simulink model "gait_recorder"  (R2015b)
settings: Solver=FixedStepDiscrete  StartTime=0.0  StopTime=inf  FixedStep=.0001  RelTol=1e-3
libraries: xpcethercatlib x14, slrtlib x8
settings Model: xpc_rtwmakecfg_data=_xpcethercatlib_  SimulationMode=external  Creator=rtheyyun  LastModifiedBy=rafae
settings SolverCC: EnableConcurrentExecution=on  ConcurrentTasks=on
settings DataIOCC: SaveFinalState=on  SaveFormat=StructureWithTime  SignalLoggingSaveFormat=ModelDataLogs  InspectSignalLogs=on
settings OptimizationCC: BlockReduction=off  OptimizeBlockIOStorage=off  BufferReuse=off  GlobalBufferReuse=off  ExpressionFolding=off  ExpressionDepthLimit=2147483647  LocalBlockOutputs=off
settings DebuggingCC: ReadBeforeWriteMsg=DisableAll  WriteAfterWriteMsg=DisableAll  WriteAfterReadMsg=DisableAll  UnderspecifiedInitializationDetection=Classic  MergeDetectMultiDrivingBlocksExec=none  SolverPrmCheckMsg=warning  InheritedTsInSrcMsg=none  FcnCallInpInsideContextMsg=UseLocalSettings  StateNameClashWarn=warning
settings HardwareCC: ProdBitPerPointer=32  ProdLargestAtomicFloat=None  ProdWordSize=32  ProdLongLongMode=on  ProdHWDeviceType=Generic->32-bit x86 compatible
settings RTWCC: SystemTargetFile=slrt.tlc  TemplateMakefile=slrt_default_tmf  Description=Simulink Real-Time  RTWVerbose=off  RTWCompilerOptimization=on
settings SimulinkRealTimeCC: GeneratePreprocessorConditionals=Disable all  xPCisModelTimeout=off  xPCModelTimeoutSecs=20  xPCConcurrentTasks=on
settings ConfigComp: CovModelRefEnable=Off  CovSFcnEnable=off

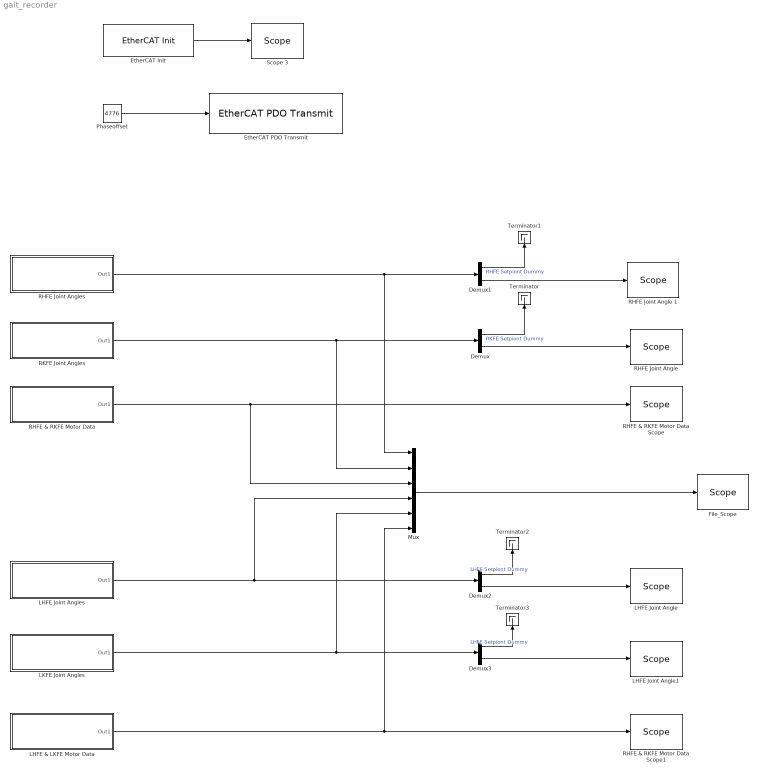
== system gait_recorder ==
  Demux{,1..3} (4 alike) : Demux  Outputs=2
  "EtherCAT Init " : xpcethercatlib/EtherCAT Init   Priority=0  config_file=C:\Users\rafae\Documents\GitHub\simulink-models\EtherCAT Config files\quad_slave_both_legs_v1.0.xml  device_id=0  pci_bus=2  pci_slot=0  dctuning=2  enaDebug=off  enaDC=off  errLink=on  masterDbg=on  stateChgDbg=on  baseClock=off  masterCfg=on  logFile='c:\dbglog.txt'  sample_time=0.001000
  "EtherCAT PDO Transmit " : xpcethercatlib/EtherCAT PDO Transmit   Priority=3  sig_name=RHFE.Outputs.jointSetpoint  sig_offset=12496  sig_type=uint32  type_size=32  sig_dim=1  device_id=0  sample_time=0.001000
  File_Scope : slrtlib/Displays and Logging/Scope   scopeno=8  scopetype=File  autostart=on  viewmode=Graphical sliding  formatstr='%15.6f'  grid=on  ylimits=[0,0]  nosamples=50000  noprepostsamples=0  interleave=1  triggermode=FreeRun  triggersignal=1  trigsignalfromport=off  triggerlevel=0.0  triggerslope=Either  triggerscope=1  triggersample=0  filename=gait.dat  mode=Lazy  writesize=512  autorestart=on  dynamicfilemode=off  maxwritefilesize=512*1024^2
  LHFE & LKFE Motor Data : Subsystem
  LHFE Joint Angle : slrtlib/Displays and Logging/Scope   scopeno=2  scopetype=Target  autostart=on  viewmode=Graphical sliding  formatstr='%15.6f'  grid=on  ylimits=[0,0]  nosamples=50000  noprepostsamples=0  interleave=1  triggermode=FreeRun  triggersignal=1  trigsignalfromport=off  triggerlevel=0.0  triggerslope=Either  triggerscope=1  triggersample=0  filename=data.dat  mode=Lazy  writesize=512  autorestart=off  dynamicfilemode=off  maxwritefilesize=512*1024^2
  LHFE Joint Angle1 : slrtlib/Displays and Logging/Scope   scopeno=5  scopetype=Target  autostart=on  viewmode=Graphical sliding  formatstr='%15.6f'  grid=on  ylimits=[0,0]  nosamples=50000  noprepostsamples=0  interleave=1  triggermode=FreeRun  triggersignal=1  trigsignalfromport=off  triggerlevel=0.0  triggerslope=Either  triggerscope=1  triggersample=0  filename=data.dat  mode=Lazy  writesize=512  autorestart=off  dynamicfilemode=off  maxwritefilesize=512*1024^2
  LHFE Joint Angles : Subsystem
  LKFE Joint Angles : Subsystem
  Mux : Mux  Inputs=6
  Phaseoffset : Constant  Value=4776  OutDataTypeStr=uint32
  RHFE & RKFE Motor Data : Subsystem
  RHFE & RKFE Motor Data Scope : slrtlib/Displays and Logging/Scope   scopeno=3  scopetype=Target  autostart=on  viewmode=Graphical sliding  formatstr='%15.6f'  grid=on  ylimits=[0,0]  nosamples=50000  noprepostsamples=0  interleave=1  triggermode=FreeRun  triggersignal=1  trigsignalfromport=off  triggerlevel=0.0  triggerslope=Either  triggerscope=1  triggersample=0  filename=data.dat  mode=Lazy  writesize=512  autorestart=off  dynamicfilemode=off  maxwritefilesize=512*1024^2
  RHFE & RKFE Motor Data Scope1 : slrtlib/Displays and Logging/Scope   scopeno=6  scopetype=Target  autostart=on  viewmode=Graphical sliding  formatstr='%15.6f'  grid=on  ylimits=[0,0]  nosamples=50000  noprepostsamples=0  interleave=1  triggermode=FreeRun  triggersignal=1  trigsignalfromport=off  triggerlevel=0.0  triggerslope=Either  triggerscope=1  triggersample=0  filename=data.dat  mode=Lazy  writesize=512  autorestart=off  dynamicfilemode=off  maxwritefilesize=512*1024^2
  "RHFE Joint Angle " : slrtlib/Displays and Logging/Scope   scopeno=4  scopetype=Target  autostart=on  viewmode=Graphical sliding  formatstr='%15.6f'  grid=on  ylimits=[0,0]  nosamples=50000  noprepostsamples=0  interleave=1  triggermode=FreeRun  triggersignal=1  trigsignalfromport=off  triggerlevel=0.0  triggerslope=Either  triggerscope=1  triggersample=0  filename=data.dat  mode=Lazy  writesize=512  autorestart=off  dynamicfilemode=off  maxwritefilesize=512*1024^2
  RHFE Joint Angle 1 : slrtlib/Displays and Logging/Scope   scopeno=1  scopetype=Target  autostart=on  viewmode=Graphical sliding  formatstr='%15.6f'  grid=on  ylimits=[0,0]  nosamples=50000  noprepostsamples=0  interleave=1  triggermode=FreeRun  triggersignal=1  trigsignalfromport=off  triggerlevel=0.0  triggerslope=Either  triggerscope=1  triggersample=0  filename=data.dat  mode=Lazy  writesize=512  autorestart=off  dynamicfilemode=off  maxwritefilesize=512*1024^2
  RHFE Joint Angles : Subsystem
  RKFE Joint Angles : Subsystem
  Scope 3 : slrtlib/Displays and Logging/Scope   scopeno=7  scopetype=Target  autostart=on  viewmode=Numerical  formatstr='%15.6f'  grid=on  ylimits=[0,0]  nosamples=3  noprepostsamples=0  interleave=1  triggermode=FreeRun  triggersignal=1  trigsignalfromport=off  triggerlevel=0.0  triggerslope=Either  triggerscope=1  triggersample=0  filename=data.dat  mode=Lazy  writesize=512  autorestart=off  dynamicfilemode=off  maxwritefilesize=512*1024^2
  Terminator{,1..3} (4 alike) : Terminator
  wires:
  "EtherCAT Init "/1 -> Scope 3/1
  Phaseoffset/1 -> "EtherCAT PDO Transmit "/1
  RHFE Joint Angles/1(Out1) -> Mux/1, Demux1/1
  Demux/2 -> "RHFE Joint Angle "/1
  Demux/1 -> Terminator/1  "RKFE Setpiont Dummy"
  RKFE Joint Angles/1(Out1) -> Mux/2, Demux/1
  Demux1/2 -> RHFE Joint Angle 1/1
  Demux1/1 -> Terminator1/1  "RHFE Setpiont Dummy"
  Mux/1 -> File_Scope/1
  RHFE & RKFE Motor Data/1(Out1) -> RHFE & RKFE Motor Data Scope/1, Mux/3
  LHFE & LKFE Motor Data/1(Out1) -> RHFE & RKFE Motor Data Scope1/1, Mux/6
  LHFE Joint Angles/1(Out1) -> Demux2/1, Mux/4
  Demux2/2 -> LHFE Joint Angle/1
  Demux2/1 -> Terminator2/1  "LHFE Setpiont Dummy"
  LKFE Joint Angles/1(Out1) -> Mux/5, Demux3/1
  Demux3/2 -> LHFE Joint Angle1/1
  Demux3/1 -> Terminator3/1  "LHFE Setpiont Dummy"

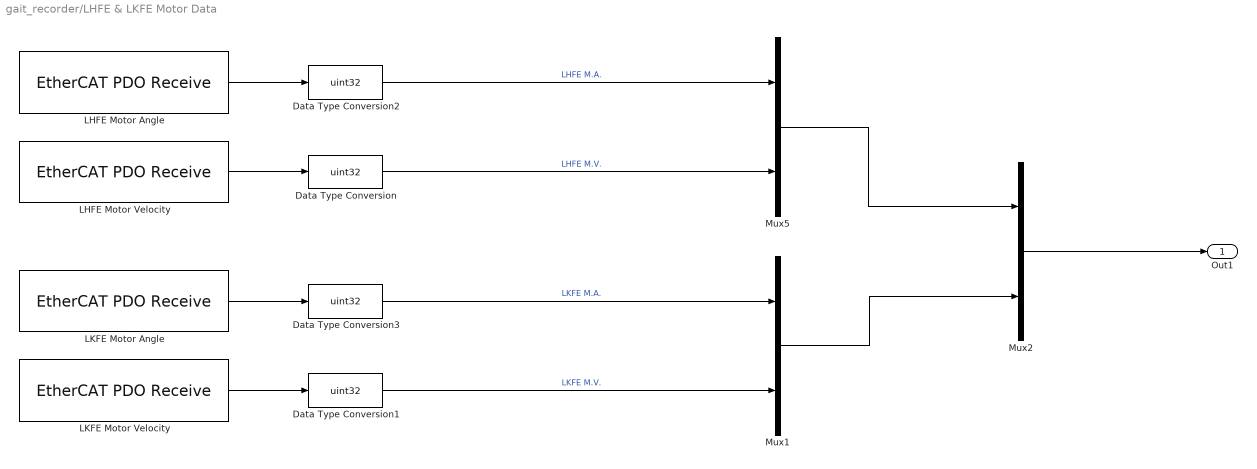
== system gait_recorder/LHFE & LKFE Motor Data ==
  Data Type Conversion{,1..3} (4 alike) : DataTypeConversion  OutDataTypeStr=uint32
  LHFE Motor Angle : xpcethercatlib/EtherCAT PDO Receive  Priority=2  sig_name=LHFE.Inputs.motorAngle  sig_offset=240  sig_type=uint16  type_size=16  sig_dim=1  device_id=0  sample_time=0.001000
  LHFE Motor Velocity : xpcethercatlib/EtherCAT PDO Receive  Priority=2  sig_name=LHFE.Inputs.motorVelocity  sig_offset=256  sig_type=int16  type_size=16  sig_dim=1  device_id=0  sample_time=0.001000
  LKFE Motor Angle : xpcethercatlib/EtherCAT PDO Receive  Priority=2  sig_name=LKFE.Inputs.motorAngle  sig_offset=528  sig_type=uint16  type_size=16  sig_dim=1  device_id=0  sample_time=0.001000
  LKFE Motor Velocity : xpcethercatlib/EtherCAT PDO Receive  Priority=2  sig_name=LKFE.Inputs.motorVelocity  sig_offset=544  sig_type=int16  type_size=16  sig_dim=1  device_id=0  sample_time=0.001000
  Mux1 : Mux  Inputs=2
  Mux2 : Mux  Inputs=2
  Mux5 : Mux  Inputs=2
  Out1 : Outport
  wires:
  Mux5/1 -> Mux2/1
  LHFE Motor Angle/1 -> Data Type Conversion2/1
  LHFE Motor Velocity/1 -> Data Type Conversion/1
  Mux1/1 -> Mux2/2
  Mux2/1 -> Out1/1
  LKFE Motor Angle/1 -> Data Type Conversion3/1
  LKFE Motor Velocity/1 -> Data Type Conversion1/1
  Data Type Conversion/1 -> Mux5/2  "LHFE M.V."
  Data Type Conversion1/1 -> Mux1/2  "LKFE M.V."
  Data Type Conversion2/1 -> Mux5/1  "LHFE M.A."
  Data Type Conversion3/1 -> Mux1/1  "LKFE M.A."

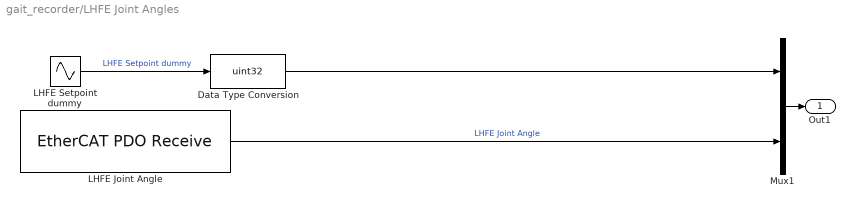
== system gait_recorder/LHFE Joint Angles ==
  Data Type Conversion : DataTypeConversion  OutDataTypeStr=uint32
  LHFE Joint Angle : xpcethercatlib/EtherCAT PDO Receive  Priority=2  sig_name=LHFE.Inputs.jointAngle  sig_offset=208  sig_type=uint32  type_size=32  sig_dim=1  device_id=0  sample_time=0.001000
  LHFE Setpoint dummy : Sin  SampleTime=0.001
  Mux1 : Mux  Inputs=2
  Out1 : Outport
  wires:
  Data Type Conversion/1 -> Mux1/1
  Mux1/1 -> Out1/1
  LHFE Joint Angle/1 -> Mux1/2  "LHFE Joint Angle"
  LHFE Setpoint dummy/1 -> Data Type Conversion/1  "LHFE Setpoint dummy"

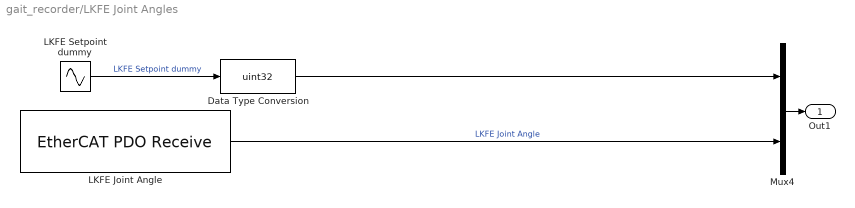
== system gait_recorder/LKFE Joint Angles ==
  Data Type Conversion : DataTypeConversion  OutDataTypeStr=uint32
  LKFE Joint Angle : xpcethercatlib/EtherCAT PDO Receive  Priority=2  sig_name=LKFE.Inputs.jointAngle  sig_offset=496  sig_type=uint32  type_size=32  sig_dim=1  device_id=0  sample_time=0.001000
  LKFE Setpoint dummy : Sin  SampleTime=0.001
  Mux4 : Mux  Inputs=2
  Out1 : Outport
  wires:
  Data Type Conversion/1 -> Mux4/1
  Mux4/1 -> Out1/1
  LKFE Joint Angle/1 -> Mux4/2  "LKFE Joint Angle"
  LKFE Setpoint dummy/1 -> Data Type Conversion/1  "LKFE Setpoint dummy"

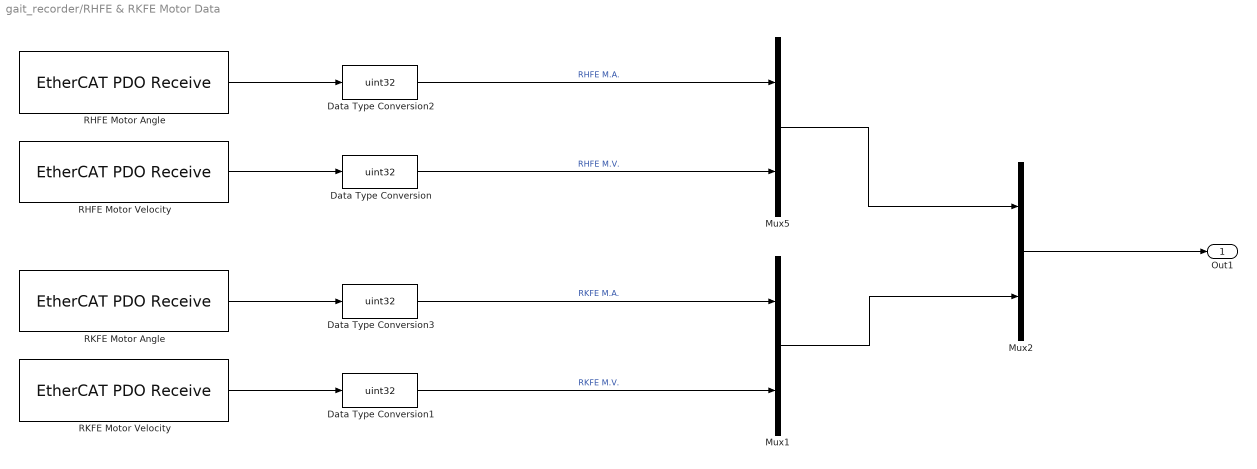
== system gait_recorder/RHFE & RKFE Motor Data ==
  Data Type Conversion{,1..3} (4 alike) : DataTypeConversion  OutDataTypeStr=uint32
  Mux1 : Mux  Inputs=2
  Mux2 : Mux  Inputs=2
  Mux5 : Mux  Inputs=2
  RHFE Motor Angle : xpcethercatlib/EtherCAT PDO Receive  Priority=2  sig_name=RHFE.Inputs.motorAngle  sig_offset=12528  sig_type=uint16  type_size=16  sig_dim=1  device_id=0  sample_time=0.001000
  RHFE Motor Velocity : xpcethercatlib/EtherCAT PDO Receive  Priority=2  sig_name=RHFE.Inputs.motorVelocity  sig_offset=12544  sig_type=int16  type_size=16  sig_dim=1  device_id=0  sample_time=0.001000
  RKFE Motor Angle : xpcethercatlib/EtherCAT PDO Receive  Priority=2  sig_name=RKFE.Inputs.motorAngle  sig_offset=12816  sig_type=uint16  type_size=16  sig_dim=1  device_id=0  sample_time=0.001000
  RKFE Motor Velocity : xpcethercatlib/EtherCAT PDO Receive  Priority=2  sig_name=RKFE.Inputs.motorVelocity  sig_offset=12832  sig_type=int16  type_size=16  sig_dim=1  device_id=0  sample_time=0.001000
  Out1 : Outport
  wires:
  Mux5/1 -> Mux2/1
  RHFE Motor Angle/1 -> Data Type Conversion2/1
  RHFE Motor Velocity/1 -> Data Type Conversion/1
  Mux1/1 -> Mux2/2
  Mux2/1 -> Out1/1
  RKFE Motor Angle/1 -> Data Type Conversion3/1
  RKFE Motor Velocity/1 -> Data Type Conversion1/1
  Data Type Conversion/1 -> Mux5/2  "RHFE M.V."
  Data Type Conversion1/1 -> Mux1/2  "RKFE M.V."
  Data Type Conversion2/1 -> Mux5/1  "RHFE M.A."
  Data Type Conversion3/1 -> Mux1/1  "RKFE M.A."

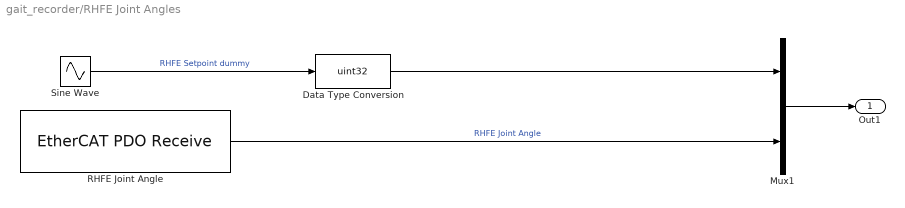
== system gait_recorder/RHFE Joint Angles ==
  Data Type Conversion : DataTypeConversion  OutDataTypeStr=uint32
  Mux1 : Mux  Inputs=2
  RHFE Joint Angle : xpcethercatlib/EtherCAT PDO Receive  Priority=2  sig_name=RHFE.Inputs.jointAngle  sig_offset=12496  sig_type=uint32  type_size=32  sig_dim=1  device_id=0  sample_time=0.001000
  Sine Wave : Sin  SampleTime=0.001
  Out1 : Outport
  wires:
  Sine Wave/1 -> Data Type Conversion/1  "RHFE Setpoint dummy"
  Mux1/1 -> Out1/1
  RHFE Joint Angle/1 -> Mux1/2  "RHFE Joint Angle"
  Data Type Conversion/1 -> Mux1/1

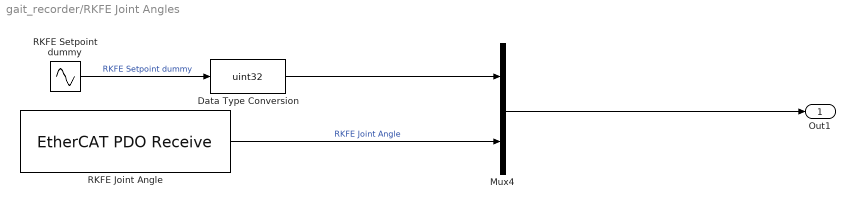
== system gait_recorder/RKFE Joint Angles ==
  Data Type Conversion : DataTypeConversion  OutDataTypeStr=uint32
  Mux4 : Mux  Inputs=2
  RKFE Joint Angle : xpcethercatlib/EtherCAT PDO Receive  Priority=2  sig_name=RKFE.Inputs.jointAngle  sig_offset=12784  sig_type=uint32  type_size=32  sig_dim=1  device_id=0  sample_time=0.001000
  RKFE Setpoint dummy : Sin  SampleTime=0.001
  Out1 : Outport
  wires:
  Data Type Conversion/1 -> Mux4/1
  Mux4/1 -> Out1/1
  RKFE Joint Angle/1 -> Mux4/2  "RKFE Joint Angle"
  RKFE Setpoint dummy/1 -> Data Type Conversion/1  "RKFE Setpoint dummy"
